simulink model "QPSK_carrier_timing_synch"  (R2014b)
settings: Solver=ode45  StartTime=0.0  StopTime=samp/fs  RelTol=1e-3
PreLoadFcn:
  | %%%%%%%%%%%%%%%%%%%%%%%%%%%%%%%%%%%%%%%%%%%%%%%%%%%%%%%%%%%%%%%%%%%%%%%%%%%
  | % check to see if Simulink library folder is missing from the MATLAB path %
  | %%%%%%%%%%%%%%%%%%%%%%%%%%%%%%%%%%%%%%%%%%%%%%%%%%%%%%%%%%%%%%%%%%%%%%%%%%%
  | if isempty(strfind(path, 'rtlsdr_book_library'))
  | 
  |     % create error window
  |     fig_error = figure(...
  |         'Name', 'Error: RTL-SDR Book Library',...
  |         'Toolbar','none',...
  |         'MenuBar','none',...
  |         'NumberTitle','off',...
  |         'Resize','off',...
  |         'WindowStyle','modal');
  |     fig_error.Position(3) = 600;
  |     fig_error.Position(4) = 150;
  |     fig_axes = axes(...
  |         'Parent',fig_error,...
  |         'Position',[0,0,1,1],...
  |         'visible','off');
  |     % error message
  |     t_title = text(.05,.8,...
  |         'MISSING DIRECTORIES',...
  |         'FontSize',11.5);
  |     t_body = text(.075,.6,...
  |         [{'Simulink cannot find the  \it{<root>}\rm / \it{rtlsdr\_book\_library}\rm  folder in the \it{MATLAB Path}\rm.'},...
  |         {'Please set the MATLAB path following the instructions given in Exercise 2.4.'}],...
  |         'FontSize',10.5);
  |     % buttons
  |     btn_path = uicontrol(...
  |         'Parent',fig_error,...
  |         'String','Set Path Now',...
  |         'FontSize',10,...
  |         'Callback', 'pathtool; close(fig_error);',...
  |         'Position', [fig_error.Position(3)/2-210, 30, 200, 30]);
  |     btn_abort = uicontrol(...
  |         'Parent',fig_error,...
  |         'String','No thanks',...
  |         'FontSize',10,...
  |         'Callback', 'close(fig_error); abort=1;',...
  |         'Position', [fig_error.Position(3)/2+10, 30, 200, 30]);
  | 
  |     % pause to allow user to interact with error box
  |     uiwait(fig_error);
  | 
  |     % abort simulation
  |     try
  |         if abort==1
  |             set_param(gcs, 'SimulationCommand', 'stop');
  |         end
  |     end
  | 
  |     % if user has set path, allow diagram to be updated
  |     if ~exist('abort','var')
  |         % create error window
  |         fig_update = figure(...
  |             'Name', 'Update Diagram',...
  |             'Toolbar','none',...
  |             'MenuBar','none',...
  |             'NumberTitle','off',...
  |             'Resize','off');
  |         fig_update.Position(3) = 400;
  |         fig_update.Position(4) = 120;
  |         fig_axes = axes(...
  |             'Parent',fig_update,...
  |             'Position',[0,0,1,1],...
  |             'visible','off');
  |         % instruction message
  |         t_body = text(.075,.7,...
  |             'Once you have set the path, update the block diagram',...
  |             'FontSize',10.5);
  |         % button
  |         btn_update = uicontrol(...
  |             'Parent',fig_update,...
  |             'String','Update Block Diagram',...
  |             'FontSize',10,...
  |             'Callback', 'set_param(gcs,''SimulationCommand'',''update''); close(gcf)',...
  |             'Position', [fig_update.Position(3)/2-100, 30, 200, 30]);
  |     end
  | 
  |     % clear error components
  |     clear('fig_error','fig_update','fig_axes','t_title','t_body','btn_path','btn_abort','btn_update','abort');
  | 
  | end
  | %%%%%%%%%%%%%%%%%%%%%%%%%%%%%%%%%%%%%%%%%%%%%%%%%%%%%%%%%%%%%%%%%%%%%%%%%%%
  | 
  | 
  | % ---------------- system parameters ------------------
  | 
  | fs = 2.4e6;
  | samp = 80000 - 1;             % stop time (number of samples in the simulation - 1)
  | 
  | Rdata = 100e3;
  | Rsymbol = Rdata/2;
  | interp = fs/Rsymbol;
  | n_sym = samp/interp;
  | fc = 400e3;                        % carrier frequency (IF modulated)
  | 
  | % ---------------- synch loop design ------------------
  | 
  | d = 0.707;                         % damping ratio (using the same for both loops)
  | 
  | % *** CARRIER synch loop *** (note this operates at symbol rate)
  | 
  | T = 1/Rsymbol;                  % sample period
  | Kp = 1;                              % phase detector S-curve is linear
  | Bn = 0.02*Rsymbol;           % bandwidth in Hz
  | Ko = 1;                              % gain of NCO
  | 
  | % calculate the loop filter coefficients for the carrier synch loop
  | K1 = (4*d*Bn*T)/(Ko*Kp*(d+1/(4*d)));
  | K2 = (4*(Bn*T)^2)/(Ko*Kp*(d+1/4*d)^2);
  | 
  | 
  | % *** SYMBOL TIMING synch loop ***
  | 
  | Ts = 1/Rsymbol;                 % symbol period
  | Ks = 3.24;                            % phase detector coefficient
  | BnS = 0.1*Rsymbol;         % bandwidth in Hz
  | Kn   = 1;                            % gain of numerically controlled clock
  | 
  | % calculate loop filter coefficients
  | Ka = (4*d*BnS*Ts)/(Kn*Ks*(d+1/(4*d)));
  | Kb = (4*(BnS*Ts)^2)/(Kn*Ks*(d+1/4*d)^2);
StopFcn:
  | % run a MATLAB script to generate some plots
  | % of the simulation results.
  | 
  | generate_receiver_plots;
undefined symbols (not defined in the file or in its folder): startfcn_constellation
libraries: simulink x5, commfilt2 x4, dsparch4 x2, commrandsrc2 x1, commdigbbndpm3 x1, rtlsdr_book_library x1
CloseFcn:
  | closefcn_model;
Description:
  | Software, Simulation Examples and Design Exercises Licence Agreement
  | 
  | This license agreement refers to the simulation examples, design exercises and files,
  | and associated software MATLAB and Simulink resources that accompany the book:
  | 
  |      Title: Software Defined Radio using MATLAB & Simulink and the RTL-SDR
  |      Published by Strathclyde Academic Media, 2015
  |      Authored by Robert W. Stewart, Kenneth W. Barlee, Dale S.W. Atkinson,
  |      and Louise H. Crockett
  | 
  | and made available as a download from, www.desktopSDR.com or variously acquired
  | by other means such as via USB storage, cloud storage, disk or any other electronic
  | or optical or magnetic storage mechanism. These files and associated software may
  | be used subject to the terms of agreement of the conditions below:
  | 
  |     Copyright © 2015 Robert W. Stewart, Kenneth W. Barlee, Dale S.W. Atkinson,
  |     and Louise H. Crockett
  |     All rights reserved.
  | 
  | Redistribution and use in source and binary forms, with or without modification, are
  | permitted provided that the following conditions are met:
  | 
  |    1.  Redistributions of source code must retain the above copyright notice, this list of
  |         conditions and the following disclaimer.
  | 
  |    2.  Redistributions in binary form must reproduce the above copyright notice, this
  |         list of conditions and the following disclaimer in the documentation and/or other
  |         materials provided with the distribution.
  | 
  |    3.  Neither the name of the copyright holder nor the names of its contributors may
  |         be used to endorse or promote products derived from this software without
  |         specific prior written permission.
  | 
  |    4.  In all cases, the software is, and all modifications and derivatives of the
  |         software shall be, licensed to you solely for use in conjunction with The
  |         MathWorks, Inc. products and service offerings.
  | 
  | THIS SOFTWARE IS PROVIDED BY THE COPYRIGHT HOLDERS AND CONTRIBUTORS
  | "AS IS" AND ANY EXPRESS OR IMPLIED WARRANTIES, INCLUDING, BUT NOT LIMITED
  | TO, THE IMPLIED WARRANTIES OF MERCHANTABILITY AND FITNESS FOR A
  | PARTICULAR PURPOSE ARE DISCLAIMED. IN NO EVENT SHALL THE COPYRIGHT
  | HOLDER OR CONTRIBUTORS BE LIABLE FOR ANY DIRECT, INDIRECT, INCIDENTAL,
  | SPECIAL, EXEMPLARY, OR CONSEQUENTIAL DAMAGES (INCLUDING, BUT NOT
  | LIMITED TO, PROCUREMENT OF SUBSTITUTE GOODS OR SERVICES; LOSS OF USE,
  | DATA, OR PROFITS; OR BUSINESS INTERRUPTION) HOWEVER CAUSED AND ON ANY
  | THEORY OF LIABILITY, WHETHER IN CONTRACT, STRICT LIABILITY, OR TORT
  | (INCLUDING NEGLIGENCE OR OTHERWISE) ARISING IN ANY WAY OUT OF THE USE
  | OF THIS SOFTWARE, EVEN IF ADVISED OF THE POSSIBILITY OF SUCH DAMAGE.
  | 
  | 
  | Audio Tracks used in Simulations Examples and Design Exercises
  | 
  | The music and vocal files used within the Examples files and software within the book
  | were variously written, arranged, performed, recorded and produced by Garrey Rice,
  | Adam Struth, Jamie Struth, Iain Thistlethwaite and also Marshall Craigmyle who
  | collectively, and individually where appropriate, assert and retain all of their copyright,
  | performance and artistic rights. Permission to use and reproduce this music is
  | granted for all purposes associated with MATLAB and Simulink software and the
  | simulation examples and design exercises files that accompany this book. Requests to
  | use the music for any other purpose should be directed to: info@desktopSDR.com.
  | For information on music track names, full credits, and links to the musicians please
  | refer to www.desktopSDR.com/more/audio.
settings Model: Creator=desktopSDR Team  LastModifiedBy=desktopSDR Team
settings DataIOCC: LimitDataPoints=off  SaveOutput=off  SignalLogging=off  SaveTime=off
settings DebuggingCC: UnderspecifiedInitializationDetection=Classic  MergeDetectMultiDrivingBlocksExec=none

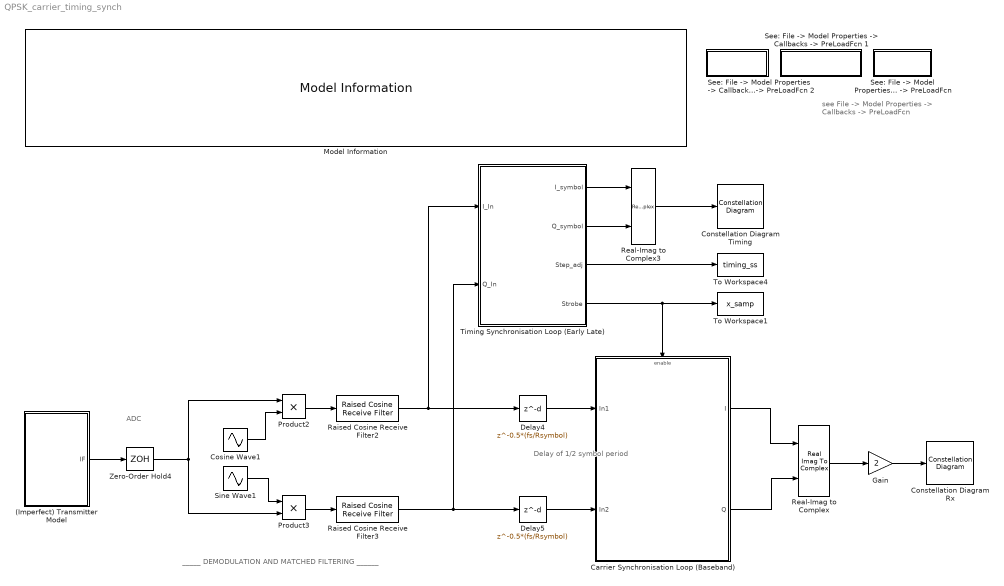
== system QPSK_carrier_timing_synch ==
  note: _____ DEMODULATION AND MATCHED FILTERING ______
  note: Delay of 1/2
      | symbol period
  note: ADC
  note: see File -> Model Properties
      | -> Callbacks -> PreLoadFcn
  (Imperfect) Transmitter Model : Subsystem  mask(Model of a QPSK Transmitter with Timing and Frequency Offsets){T_error=50, F_error=-200}
      mask prompts: T_error "Timing Error (ppm)"; F_error "Frequency Error (Hz)"
      mask help:
      | Enter the timing and frequency offsets that apply to the received signal.
      |
      | Both of these can be negative or positive values. Negative means that the timing / frequency of the transmitter is lower than expected.
      mask init:
      | T_Offset = 1+(T_error/1e6);
      | F_Offset = F_error;
  Carrier Synchronisation Loop (Baseband) : Subsystem
  Constellation Diagram Rx : ConstellationDiagram  StartFcn=startfcn_constellation;
  Constellation Diagram Timing : ConstellationDiagram  StartFcn=startfcn_constellation;
  Cosine Wave1 : Sin  Amplitude=sqrt(2)  Frequency=fc*2*pi  Phase=pi/2  SampleTime=1/fs
  Delay4 : Delay  DelayLength=0.5*(fs/Rsymbol)
  Delay5 : Delay  DelayLength=0.5*(fs/Rsymbol)
  Gain : Gain  Gain=2
  Model Information : rtlsdr_book_library/Additional Tools/Model Information/Model Information
  Product2 : Product
  Product3 : Product
  Raised Cosine Receive Filter2 : commfilt2/Raised Cosine Receive Filter  filtType=Square root  N=interp  filtSpan=12  currentFiltSpan=12  D=(12)/2  R=0.35  sampMode=Mute  saveAsFlag=0  rateMode=Downsampling  downFactor=1  downOffset=0  framing=Allow multirate processing  checkGain=Normalized  filterGain=1  checkCoeff=off  variableName=rcRxFilt2  launchFVT=on  roundingMode=Floor  overflowMode=off
  Raised Cosine Receive Filter3 : commfilt2/Raised Cosine Receive Filter  filtType=Square root  N=interp  filtSpan=12  currentFiltSpan=12  D=(12)/2  R=0.35  sampMode=Mute  saveAsFlag=0  rateMode=Downsampling  downFactor=1  downOffset=0  framing=Allow multirate processing  checkGain=Normalized  filterGain=1  checkCoeff=off  variableName=rcRxFilt3  launchFVT=on  roundingMode=Floor  overflowMode=off
  Real-Imag to Complex : RealImagToComplex
  Real-Imag to Complex3 : RealImagToComplex
  "See: File -> Model Properties -> Callbacks -> PreLoadFcn " : Subsystem
      mask Display:
      | fs = evalin('base', 'fs');
      | fprintf(['fs = ',num2str(fs/1e6),' MHz']);
  "See: File -> Model Properties -> Callbacks -> PreLoadFcn 1" : Subsystem
      mask Display:
      | Rsymbol = evalin('base', 'Rsymbol');
      | fprintf(['Rsymbol = ',num2str(Rsymbol/1e3),' ksps']);
  "See: File -> Model Properties -> Callbacks -> PreLoadFcn 2" : Subsystem
      mask Display:
      | Rsymbol = evalin('base', 'Rsymbol');
      | fs = evalin('base', 'fs');
      | fprintf(['OSR = ',num2str(fs/Rsymbol)]);
  Sine Wave1 : Sin  Amplitude=sqrt(2)  Frequency=fc*2*pi  SampleTime=1/fs
  Timing Synchronisation Loop (Early Late) : Subsystem  mask(Early Late Timing Error Detector){OSR=fs/Rsymbol, Ka=Ka, Kb=Kb}
      mask prompts: OSR "Oversampling ratio (even integer value)"; Ka "Ka (Loop Filter proportial gain)"; Kb "Kb (Loop Filter integral gain)"
      mask help:
      | This TED works with quadrature (I and Q) inputs and generates a strobe for sampling the punctual branch at the optimal timing instants.
      |
      | The model can be parameterised in terms of the oversampling ratio and the design of the timing PLL.
      |
      | Note that the oversampling ratio must be an EVEN INTEGER value.
  To Workspace1 : ToWorkspace  VariableName=x_samp  SaveFormat=Structure With Time  SampleTime=1/fs
  To Workspace4 : ToWorkspace  VariableName=timing_ss  SaveFormat=Structure With Time  SampleTime=1/fs
  Zero-Order Hold4 : ZeroOrderHold  SampleTime=1/fs
  wires:
  Real-Imag to Complex/1 -> Gain/1
  Gain/1 -> Constellation Diagram Rx/1
  Cosine Wave1/1 -> Product2/2
  Sine Wave1/1 -> Product3/1
  Carrier Synchronisation Loop (Baseband)/1(I) -> Real-Imag to Complex/1
  Carrier Synchronisation Loop (Baseband)/2(Q) -> Real-Imag to Complex/2
  Delay4/1 -> Carrier Synchronisation Loop (Baseband)/1(In1)
  Delay5/1 -> Carrier Synchronisation Loop (Baseband)/2(In2)
  Product2/1 -> Raised Cosine Receive Filter2/1
  Product3/1 -> Raised Cosine Receive Filter3/1
  Raised Cosine Receive Filter2/1 -> Timing Synchronisation Loop (Early Late)/1(I_In), Delay4/1
  Raised Cosine Receive Filter3/1 -> Delay5/1, Timing Synchronisation Loop (Early Late)/2(Q_In)
  Zero-Order Hold4/1 -> Product2/1, Product3/2
  (Imperfect) Transmitter Model/1(IF) -> Zero-Order Hold4/1
  Timing Synchronisation Loop (Early Late)/4(Strobe) -> To Workspace1/1, Carrier Synchronisation Loop (Baseband)/Enable
  Timing Synchronisation Loop (Early Late)/1(I_symbol) -> Real-Imag to Complex3/1
  Timing Synchronisation Loop (Early Late)/2(Q_symbol) -> Real-Imag to Complex3/2
  Real-Imag to Complex3/1 -> Constellation Diagram Timing/1
  Timing Synchronisation Loop (Early Late)/3(Step_adj) -> To Workspace4/1

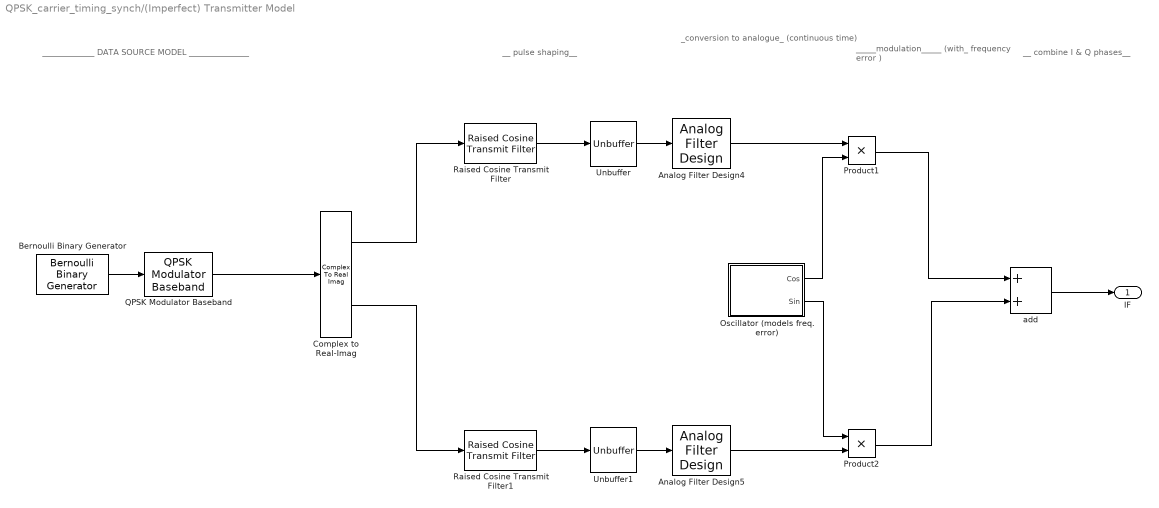
== system QPSK_carrier_timing_synch/(Imperfect) Transmitter Model ==
  note: _____________ DATA SOURCE MODEL _______________
  note: _conversion to analogue_
      | (continuous time)
  note: __ pulse shaping__
  note: _____modulation_____
      | (with_ frequency error )
  note: __ combine I & Q phases__
  Analog Filter Design4 : dsparch4/Analog Filter Design  method=Butterworth  filttype=Lowpass  N=8  Wlo=2*pi*Rsymbol*T_Offset  Whi=80  Rp=2  Rs=40
  Analog Filter Design5 : dsparch4/Analog Filter Design  method=Butterworth  filttype=Lowpass  N=8  Wlo=2*pi*Rsymbol*T_Offset  Whi=80  Rp=2  Rs=40
  Bernoulli Binary Generator : commrandsrc2/Bernoulli Binary Generator  P=0.5  seed=61  Ts=1/(T_Offset*Rdata)  frameBased=on  sampPerFrame=2  orient=off  outDataType=double
  Complex to Real-Imag : ComplexToRealImag
  Oscillator (models freq. error) : Subsystem
  Product1 : Product
  Product2 : Product
  QPSK Modulator Baseband : commdigbbndpm3/QPSK Modulator Baseband  InType=Bit  Enc=Gray  Ph=pi/4  outDtype=double  outWordLen=16  outUDDataType=sfix(16)  outFracLenMode=Best precision  outFracLen=15
  Raised Cosine Transmit Filter : commfilt2/Raised Cosine Transmit Filter  filtType=Square root  filtSpan=12  currentFiltSpan=12  D=(12)/2  R=0.35  sampMode=Mute  saveAsFlag=0  N=fs/Rsymbol  framing=Allow multirate processing  InputProcessing=Columns as channels (frame based)  checkGain=Normalized  filterGain=1  checkCoeff=off  variableName=rcTxFilt  launchFVT=on  roundingMode=Floor  overflowMode=off
  Raised Cosine Transmit Filter1 : commfilt2/Raised Cosine Transmit Filter  filtType=Square root  filtSpan=12  currentFiltSpan=12  D=(12)/2  R=0.35  sampMode=Mute  saveAsFlag=0  N=fs/Rsymbol  framing=Allow multirate processing  InputProcessing=Columns as channels (frame based)  checkGain=Normalized  filterGain=1  checkCoeff=off  variableName=rcTxFilt1  launchFVT=on  roundingMode=Floor  overflowMode=off
  Unbuffer : Unbuffer  SampleBasedProcessing=Same as frame based
  Unbuffer1 : Unbuffer  SampleBasedProcessing=Same as frame based
  add : Sum
  IF : Outport
  wires:
  Raised Cosine Transmit Filter1/1 -> Unbuffer1/1
  Complex to Real-Imag/2 -> Raised Cosine Transmit Filter1/1
  Complex to Real-Imag/1 -> Raised Cosine Transmit Filter/1
  Bernoulli Binary Generator/1 -> QPSK Modulator Baseband/1
  Raised Cosine Transmit Filter/1 -> Unbuffer/1
  Product1/1 -> add/1
  Analog Filter Design4/1 -> Product1/1
  Analog Filter Design5/1 -> Product2/2
  Product2/1 -> add/2
  add/1 -> IF/1
  Oscillator (models freq. error)/1(Cos) -> Product1/2
  Oscillator (models freq. error)/2(Sin) -> Product2/1
  QPSK Modulator Baseband/1 -> Complex to Real-Imag/1
  Unbuffer/1 -> Analog Filter Design4/1
  Unbuffer1/1 -> Analog Filter Design5/1

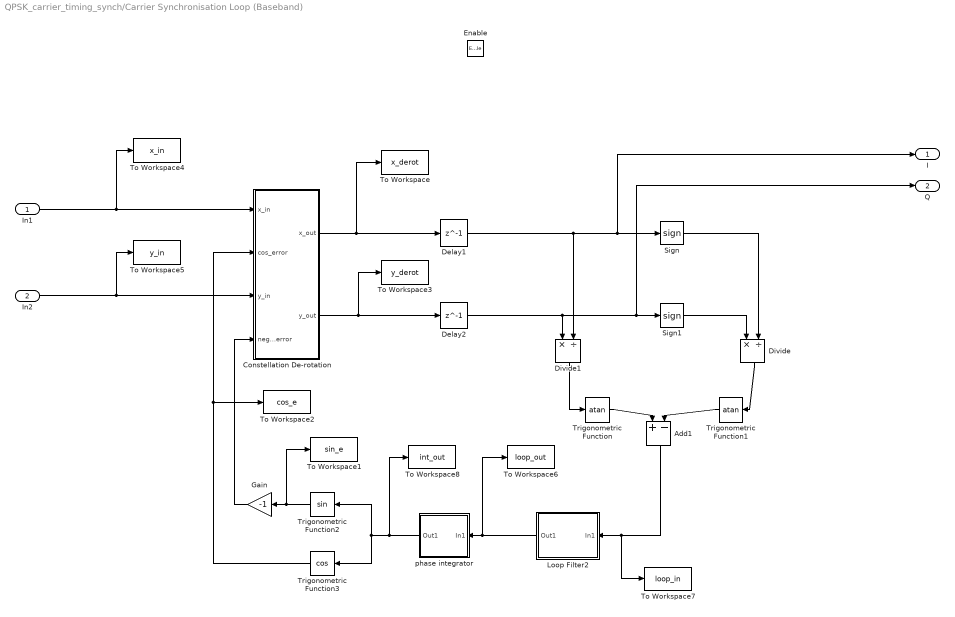
== system QPSK_carrier_timing_synch/Carrier Synchronisation Loop (Baseband) ==
  In1 : Inport
  In2 : Inport  Port=2
  Enable : EnablePort
  Add1 : Sum  Inputs=+-
  Constellation De-rotation : Subsystem
  Delay1 : Delay  DelayLength=1  InitialCondition=1
  Delay2 : Delay  DelayLength=1  InitialCondition=0
  Divide : Product  Inputs=*/
  Divide1 : Product  Inputs=*/
  Gain : Gain  Gain=-1
  Loop Filter2 : Subsystem
  Sign : Signum
  Sign1 : Signum
  To Workspace : ToWorkspace  VariableName=x_derot  SaveFormat=Structure With Time  SampleTime=1/fs
  To Workspace1 : ToWorkspace  VariableName=sin_e  SaveFormat=Structure With Time  SampleTime=1/fs
  To Workspace2 : ToWorkspace  VariableName=cos_e  SaveFormat=Structure With Time  SampleTime=1/fs
  To Workspace3 : ToWorkspace  VariableName=y_derot  SaveFormat=Structure With Time  SampleTime=1/fs
  To Workspace4 : ToWorkspace  VariableName=x_in  SaveFormat=Structure With Time  SampleTime=1/fs
  To Workspace5 : ToWorkspace  VariableName=y_in  SaveFormat=Structure With Time  SampleTime=1/fs
  To Workspace6 : ToWorkspace  VariableName=loop_out  SaveFormat=Structure With Time  SampleTime=-1
  To Workspace7 : ToWorkspace  VariableName=loop_in  SaveFormat=Structure With Time  SampleTime=-1
  To Workspace8 : ToWorkspace  VariableName=int_out  SaveFormat=Structure With Time  SampleTime=-1
  Trigonometric Function : Trigonometry  Operator=atan  OutputSignalType=real
  Trigonometric Function1 : Trigonometry  Operator=atan  OutputSignalType=real
  Trigonometric Function2 : Trigonometry
  Trigonometric Function3 : Trigonometry  Operator=cos
  phase integrator : Subsystem
  I : Outport
  Q : Outport  Port=2
  wires:
  Delay1/1 -> Divide1/2, I/1, Sign/1
  Sign/1 -> Divide/2
  Sign1/1 -> Divide/1
  Trigonometric Function/1 -> Add1/1
  Trigonometric Function1/1 -> Add1/2
  Trigonometric Function2/1 -> To Workspace1/1, Gain/1
  Constellation De-rotation/1(x_out) -> To Workspace/1, Delay1/1
  Divide/1 -> Trigonometric Function1/1
  Divide1/1 -> Trigonometric Function/1
  Loop Filter2/1(Out1) -> phase integrator/1(In1), To Workspace6/1
  Constellation De-rotation/2(y_out) -> To Workspace3/1, Delay2/1
  Delay2/1 -> Divide1/1, Q/1, Sign1/1
  In1/1 -> To Workspace4/1, Constellation De-rotation/1(x_in)
  In2/1 -> To Workspace5/1, Constellation De-rotation/3(y_in)
  Add1/1 -> Loop Filter2/1(In1), To Workspace7/1
  phase integrator/1(Out1) -> Trigonometric Function2/1, Trigonometric Function3/1, To Workspace8/1
  Trigonometric Function3/1 -> To Workspace2/1, Constellation De-rotation/2(cos_error)
  Gain/1 -> Constellation De-rotation/4(neg_sin_error)

== system QPSK_carrier_timing_synch/See: File -> Model Properties -> Callbacks -> PreLoadFcn  ==

== system QPSK_carrier_timing_synch/See: File -> Model Properties -> Callbacks -> PreLoadFcn 1 ==

== system QPSK_carrier_timing_synch/See: File -> Model Properties -> Callbacks -> PreLoadFcn 2 ==

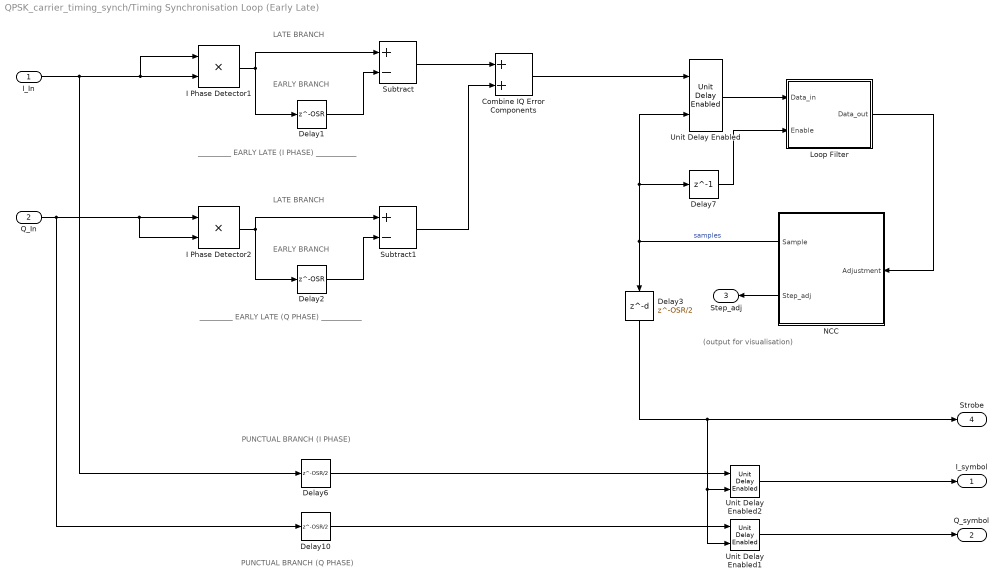
== system QPSK_carrier_timing_synch/Timing Synchronisation Loop (Early Late) ==
  note: (output for
      | visualisation)
  note: LATE BRANCH
  note: EARLY BRANCH
  note: LATE BRANCH
  note: EARLY BRANCH
  note: _________ EARLY LATE (I PHASE) ___________
  note: _________ EARLY LATE (Q PHASE) ___________
  note: PUNCTUAL BRANCH (I PHASE)
  note: PUNCTUAL BRANCH (Q PHASE)
  I_In : Inport
  Q_In : Inport  Port=2
  Combine IQ Error Components : Sum
  Delay1 : Delay  DelayLength=OSR
  Delay10 : Delay  DelayLength=OSR/2
  Delay2 : Delay  DelayLength=OSR
  Delay3 : Delay  DelayLength=OSR/2
  Delay6 : Delay  DelayLength=OSR/2
  Delay7 : Delay  DelayLength=1
  I Phase Detector1 : Product
  I Phase Detector2 : Product
  Loop Filter : Subsystem
  NCC : Subsystem  mask(Numerically Controller Clock (NCC)){OSR=OSR}
      mask prompts: OSR "Oversampling Ratio"
      mask help:
      | This component operates similarly to a Numerically Controlled Oscillator (NCO).
      |
      | Internally, a nominal step size of (1 + Adjustment) is applied to an accumulator. The accumulator wraps around at N = OSR, therefore for a zero control input, the accumulator wraps once every symbol period at the expected rate.
      |
      | When the accumulator wraps, a strobe output is produced.
  Subtract : Sum  Inputs=+-
  Subtract1 : Sum  Inputs=+-
  Unit Delay Enabled : simulink/Additional Math & Discrete/Additional Discrete/Unit Delay Enabled  vinit=0.0  tsamp=-1
  Unit Delay Enabled1 : simulink/Additional Math & Discrete/Additional Discrete/Unit Delay Enabled  vinit=0.0  tsamp=-1
  Unit Delay Enabled2 : simulink/Additional Math & Discrete/Additional Discrete/Unit Delay Enabled  vinit=0.0  tsamp=-1
  I_symbol : Outport
  Q_symbol : Outport  Port=2
  Step_adj : Outport  Port=3
  Strobe : Outport  Port=4
  wires:
  Delay2/1 -> Subtract1/2
  Subtract1/1 -> Combine IQ Error Components/2
  Unit Delay Enabled/1 -> Loop Filter/1(Data_in)
  Combine IQ Error Components/1 -> Unit Delay Enabled/1
  I Phase Detector1/1 -> Subtract/1, Delay1/1
  Delay1/1 -> Subtract/2
  NCC/1(Sample) -> Unit Delay Enabled/2, Delay7/1, Delay3/1  "samples"
  Subtract/1 -> Combine IQ Error Components/1
  I Phase Detector2/1 -> Delay2/1, Subtract1/1
  Loop Filter/1(Data_out) -> NCC/1(Adjustment)
  Delay7/1 -> Loop Filter/2(Enable)
  NCC/2(Step_adj) -> Step_adj/1
  Q_In/1 -> Delay10/1, I Phase Detector2/2, I Phase Detector2/1
  I_In/1 -> Delay6/1, I Phase Detector1/1, I Phase Detector1/2
  Delay6/1 -> Unit Delay Enabled2/1
  Delay10/1 -> Unit Delay Enabled1/1
  Delay3/1 -> Strobe/1, Unit Delay Enabled1/2, Unit Delay Enabled2/2
  Unit Delay Enabled2/1 -> I_symbol/1
  Unit Delay Enabled1/1 -> Q_symbol/1

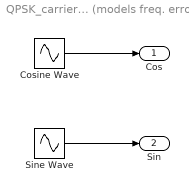
== system QPSK_carrier_timing_synch/(Imperfect) Transmitter Model/Oscillator (models freq. error) ==
  Cosine Wave : Sin  Frequency=2*pi*(fc+F_Offset)  Phase=pi/2  SampleTime=0
  Sine Wave : Sin  Frequency=2*pi*(fc+F_Offset)  SampleTime=0
  Cos : Outport
  Sin : Outport  Port=2
  wires:
  Sine Wave/1 -> Sin/1
  Cosine Wave/1 -> Cos/1

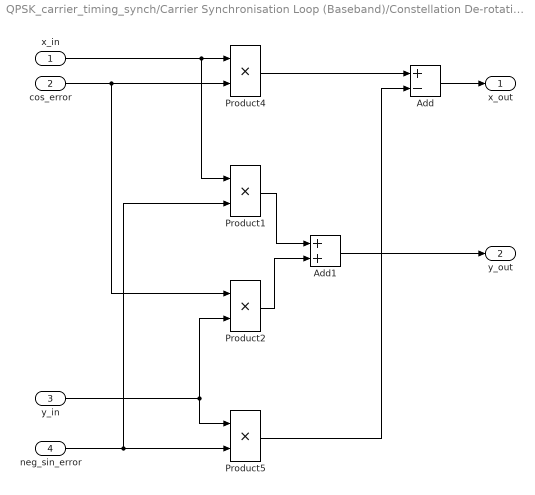
== system QPSK_carrier_timing_synch/Carrier Synchronisation Loop (Baseband)/Constellation De-rotation ==
  x_in : Inport
  cos_error : Inport  Port=2
  y_in : Inport  Port=3
  neg_sin_error : Inport  Port=4
  Add : Sum  Inputs=+-
  Add1 : Sum
  Product{1..2,4..5} (4 alike) : Product
  x_out : Outport
  y_out : Outport  Port=2
  wires:
  Product4/1 -> Add/1
  Product5/1 -> Add/2
  cos_error/1 -> Product2/1, Product4/2
  Add/1 -> x_out/1
  neg_sin_error/1 -> Product5/2, Product1/2
  Product2/1 -> Add1/2
  Product1/1 -> Add1/1
  Add1/1 -> y_out/1
  y_in/1 -> Product5/1, Product2/2
  x_in/1 -> Product4/1, Product1/1

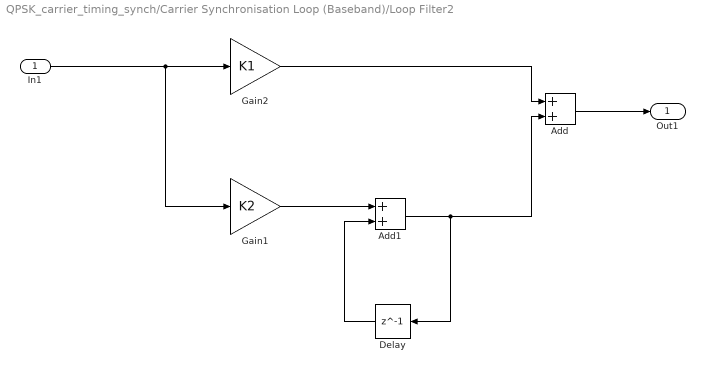
== system QPSK_carrier_timing_synch/Carrier Synchronisation Loop (Baseband)/Loop Filter2 ==
  In1 : Inport
  Add : Sum
  Add1 : Sum
  Delay : Delay  DelayLength=1  InitialCondition=0
  Gain1 : Gain  Gain=K2
  Gain2 : Gain  Gain=K1
  Out1 : Outport
  wires:
  Gain1/1 -> Add1/1
  Add/1 -> Out1/1
  Gain2/1 -> Add/1
  Delay/1 -> Add1/2
  Add1/1 -> Delay/1, Add/2
  In1/1 -> Gain1/1, Gain2/1

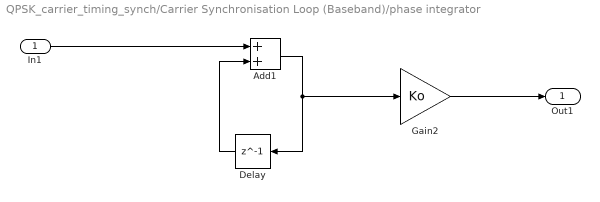
== system QPSK_carrier_timing_synch/Carrier Synchronisation Loop (Baseband)/phase integrator ==
  In1 : Inport
  Add1 : Sum
  Delay : Delay  DelayLength=1  InitialCondition=0
  Gain2 : Gain  Gain=Ko
  Out1 : Outport
  wires:
  In1/1 -> Add1/1
  Add1/1 -> Delay/1, Gain2/1
  Delay/1 -> Add1/2
  Gain2/1 -> Out1/1

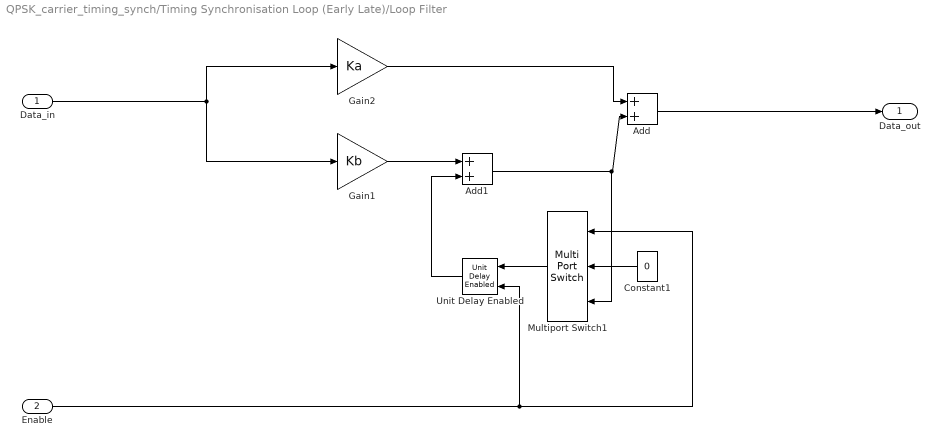
== system QPSK_carrier_timing_synch/Timing Synchronisation Loop (Early Late)/Loop Filter ==
  Data_in : Inport
  Enable : Inport  Port=2
  Add : Sum
  Add1 : Sum
  Constant1 : Constant  Value=0  SampleTime=1/fs
  Gain1 : Gain  Gain=Kb
  Gain2 : Gain  Gain=Ka
  Multiport Switch1 : MultiPortSwitch  DataPortOrder=Zero-based contiguous  Inputs=2
  Unit Delay Enabled : simulink/Additional Math & Discrete/Additional Discrete/Unit Delay Enabled  vinit=0.0  tsamp=-1
  Data_out : Outport
  wires:
  Gain1/1 -> Add1/1
  Gain2/1 -> Add/1
  Unit Delay Enabled/1 -> Add1/2
  Add1/1 -> Multiport Switch1/3, Add/2
  Data_in/1 -> Gain2/1, Gain1/1
  Add/1 -> Data_out/1
  Enable/1 -> Unit Delay Enabled/2, Multiport Switch1/1
  Multiport Switch1/1 -> Unit Delay Enabled/1
  Constant1/1 -> Multiport Switch1/2

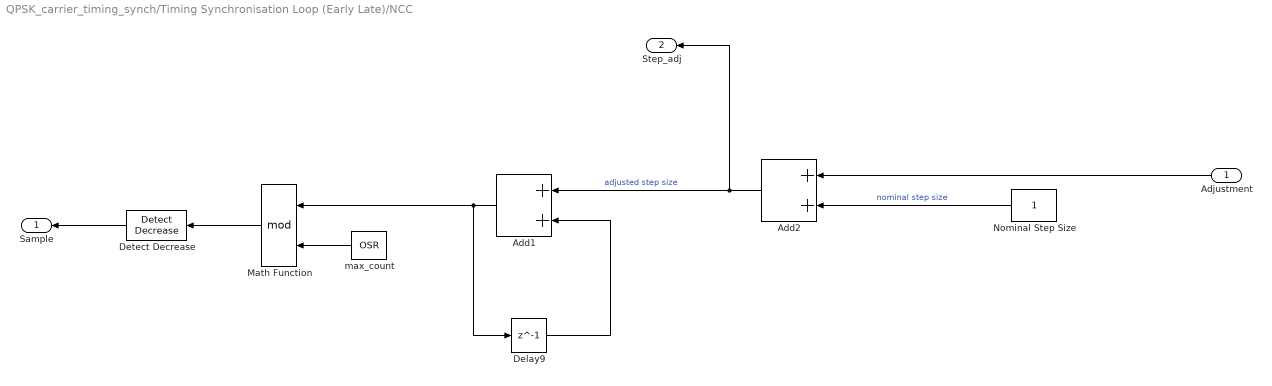
== system QPSK_carrier_timing_synch/Timing Synchronisation Loop (Early Late)/NCC ==
  Adjustment : Inport
  Add1 : Sum  OutDataTypeStr=double
  Add2 : Sum  OutDataTypeStr=double
  Delay9 : Delay  DelayLength=1
  Detect Decrease : simulink/Logic and Bit Operations/Detect Decrease  vinit=0.0  InputProcessing=Inherited  OutDataTypeStr=boolean
  Math Function : Math  Operator=mod  SaturateOnIntegerOverflow=on
  Nominal Step Size : Constant  OutDataTypeStr=double  SampleTime=1/fs
  max_count : Constant  Value=OSR  OutDataTypeStr=double  SampleTime=1/fs
  Sample : Outport
  Step_adj : Outport  Port=2
  wires:
  Adjustment/1 -> Add2/1
  Add2/1 -> Step_adj/1, Add1/1  "adjusted step size"
  Delay9/1 -> Add1/2
  Nominal Step Size/1 -> Add2/2  "nominal step size"
  Add1/1 -> Delay9/1, Math Function/1
  Math Function/1 -> Detect Decrease/1
  max_count/1 -> Math Function/2
  Detect Decrease/1 -> Sample/1
